simulink model "gtcs_math_v1"  (R2022b)
settings: Solver=VariableStepAuto  StartTime=0.0  StopTime=10  RelTol=1e-3
values from neighbouring files (symbols this model uses):
  B_load = 0.0047    [parameter_andar_servomotor.mat]
  B_motor = 0.00025    [parameter_andar_servomotor.mat]    (also in parameter_original_servomotor.mat)
  B_reducer = 0.001    [parameter_andar_servomotor.mat]
  GearRatio = 1    [parameter_andar_servomotor.mat]
  J_hysteresis_brake = 0.0016118    [parameter_andar_servomotor.mat]
  J_load = 0.0016118    [parameter_andar_servomotor.mat]
  J_motor = 0.0002548    [parameter_andar_servomotor.mat]    (also in parameter_original_servomotor.mat = 0.001)
  J_reducer = 1e-05    [parameter_andar_servomotor.mat]
  ke = 0.039313695    [parameter_andar_servomotor.mat]    (also in parameter_original_servomotor.mat = 0.04001501117)
  kt = 0.0378    [parameter_andar_servomotor.mat]    (also in parameter_original_servomotor.mat = 0.0375)
  L_motor = 6e-06    [parameter_andar_servomotor.mat]    (also in parameter_original_servomotor.mat = 3e-05)
  R_motor = 0.015    [parameter_andar_servomotor.mat]    (also in parameter_original_servomotor.mat = 0.075)
undefined symbols (not defined in the file or in its folder): sigbuilder_block
libraries: simulink x3, slpidlib x1
settings Model: DataDictionary=gtcs_math_v1.sldd  Creator=yusuf.ogut  LastModifiedBy=Yusuf
settings ModelReferenceCC: EnableRefExpFcnMdlSchedulingChecks=on

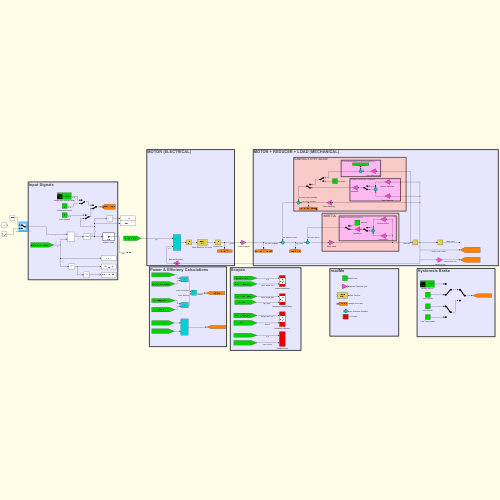
[thumbnail: Simulink's stored preview of the top-level diagram]
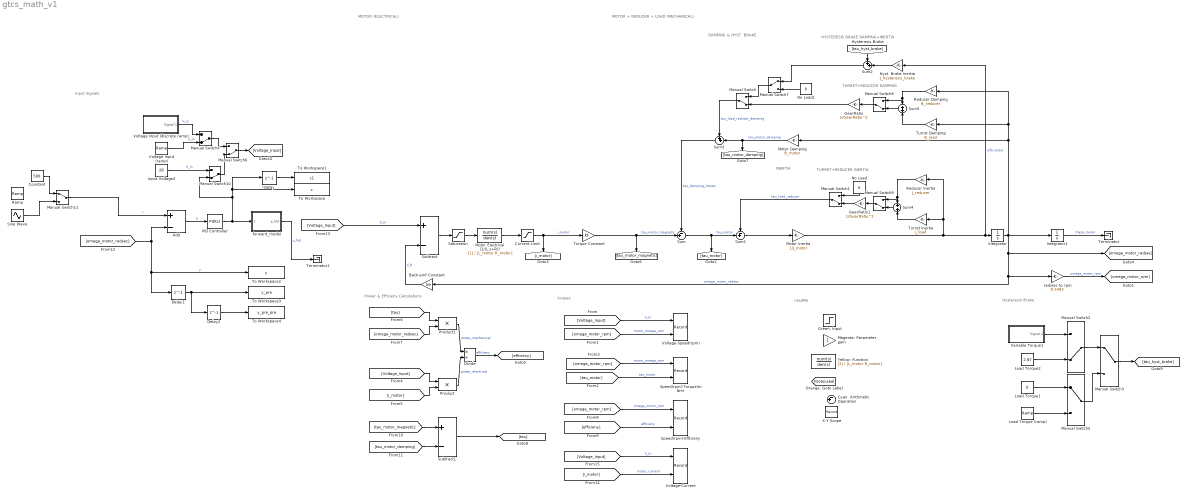
== system gtcs_math_v1 ==
  note: TURRET+REDUCER INERTIA
  note: TURRET+REDUCER DAMPING
  note: HYSTERESIS BRAKE DAMPING+INERTIA
  note: DAMPING & HYST. BRAKE
  note: INERTIA
  note: readMe
  note: MOTOR (ELECTRICAL)
  note: MOTOR + REDUCER + LOAD (MECHANICAL)
  note: Hysteresis Brake
  note: Input Signals
  note: Scopes
  note: Power & Efficieny Calculations
  Add : Sum  Inputs=+-
  Back-emf Constant : Gain  Gain=ke
  Constant : Constant  Value=500
  Current Limit : Saturate  UpperLimit=80  LowerLimit=-80
  Cyan: Arithmetic Operation : Sum  Inputs=-+|
  Delay : Delay  DelayLength=1  SampleTime=0.01
  Delay1 : Delay  DelayLength=1  SampleTime=0.01
  Delay2 : Delay  DelayLength=1  SampleTime=0.01
  Divide : Product  Inputs=*/
  GearRatio : Gain  Gain=1/GearRatio^2
  GearRatio1 : Gain  Gain=1/GearRatio^2
  Green: Input : Step  SampleTime=0
  Hyst. Brake Inertia : Gain  Gain=J_hysteresis_brake
  Input Voltage2 : Constant  Value=28
  Integrator : Integrator
  Integrator1 : Integrator
  Load Torque (ramp) : simulink/Sources/Ramp  slope=2.9/27  start=0  InitialOutput=1e-06
  Load Torque1 : Constant  Value=0
  Load Torque2 : Constant  Value=2.87
  "Magenta: Parameter, gain" : Gain
  Manual Switch{,1..2,4,6,8..10} (8 alike) : ManualSwitch  CurrentSetting=0
  Manual Switch{3,5,7,11} (4 alike) : ManualSwitch
  Motor Damping : Gain  Gain=B_motor
  Motor Electrical (1/(L.s+R)) : TransferFcn  Denominator=[L_motor R_motor]
  Motor Inertia : Gain  Gain=1/J_motor
  No Load : Constant  Value=0
  No Load1 : Constant  Value=0
  PID Controller : slpidlib/PID Controller  Controller=PID  Form=Parallel  TimeDomain=Continuous-time  UseExternalTs=off  SampleTime=-1  IntegratorMethod=Forward Euler  FilterMethod=Forward Euler  ControllerParametersSource=internal  P=1  I=1  UseKiTs=off  D=0  N=100  UseFilter=on  TunerSelectOption=Transfer Function Based (PID Tuner App)  InitialConditionSource=internal  InitialConditionForIntegrator=0  InitialConditionForFilter=0  DifferentiatorICPrevScaledInput=0  ExternalReset=none  TrackingMode=off  Kt=1  LimitOutput=off  SatLimitsSource=internal  UpperSaturationLimit=inf  LowerSaturationLimit=-inf  LinearizeAsGain=on  AntiWindupMode=none  Kb=1  LimitIntegrator=off  UpperIntegratorSaturationLimit=inf  LowerIntegratorSaturationLimit=-inf  POutMin=[]  POutMax=[]  IOutMin=[]  IOutMax=[]  DOutMin=[]  DOutMax=[]  NOutMin=[]  NOutMax=[]  SumOutMin=[]  SumOutMax=[]  SaturationOutMin=[]  SaturationOutMax=[]  PParamMin=[]  PParamMax=[]  IParamMin=[]  IParamMax=[]  DParamMin=[]  DParamMax=[]  NParamMin=[]  NParamMax=[]  KbParamMin=[]  KbParamMax=[]  KtParamMin=[]  KtParamMax=[]  KbOutMin=[]  KbOutMax=[]  KtOutMin=[]  KtOutMax=[]  IntegratorOutMin=[]  IntegratorOutMax=[]  FilterOutMin=[]  FilterOutMax=[]  SumI1OutMin=[]  SumI1OutMax=[]  SumI2OutMin=[]  SumI2OutMax=[]  SumI3OutMin=[]  SumI3OutMax=[]  SumI4OutMin=[]  SumI4OutMax=[]  SumDOutMin=[]  SumDOutMax=[]  DifferentiatorOutMin=[]  DifferentiatorOutMax=[]  FilterDiffOutCoefMin=[]  FilterDiffOutCoefMax=[]  ReciprocalOutMin=[]  ReciprocalOutMax=[]  SumDenOutMin=[]  SumDenOutMax=[]  SumNumOutMin=[]  SumNumOutMax=[]  DivideOutMin=[]  DivideOutMax=[]  UdiffTsProdOutMin=[]  UdiffTsProdOutMax=[]  NTsProdOutMin=[]  NTsProdOutMax=[]  UintegralTsProdOutMin=[]  UintegralTsProdOutMax=[]  UngainTsProdOutMin=[]  UngainTsProdOutMax=[]  ClampingZeroOutDataTypeStr=Inherit: Inherit via back propagation  ClampingZeroOutMin=[]  ClampingZeroOutMax=[]  FilterDenConstantOutDataTypeStr=Inherit: Inherit via back propagation  FilterDenConstantOutMin=[]  FilterDenConstantOutMax=[]  PCopyOutDataTypeStr=Inherit: Inherit via back propagation  PCopyOutMin=[]  PCopyOutMax=[]  NCopyOutDataTypeStr=Inherit: Inherit via back propagation  NCopyOutMin=[]  NCopyOutMax=[]  IntegratorContinuousStateAttributes=''  IntegratorStateMustResolveToSignalObject=off  IntegratorRTWStateStorageClass=Auto  FilterContinuousStateAttributes=''  FilterStateMustResolveToSignalObject=off  FilterRTWStateStorageClass=Auto  ParallelPVariant=InternalParameters  IdealPVariant=Disabled  IVariant=InternalParameters  DVariant=InternalParameters  IntegratorVariant=Continuous  SatVariant=Disabled  AWVariant=Passthrough  PCopyVariant=Disabled  TRVariant=Disabled  FdbkBlocksVariant=Forward  IdealPFdbkVariant=Disabled  SatFdbkVariant=Disabled  DerivativeFilterVariant=ContFilter  NVariant=InternalParameters  NCopyVariant=Disabled  FilterICVariant=InternalICsFilter  IntegratorICVariant=InternalICs  ExternalResetVariant=Disabled  TRSumVariant=Passthrough  SumFdbkVariant=Disabled  SumVariant=Sum_PID  TsampFilterVariant=InternalTs  TsampNgainVariant=Passthrough  TsampIntegralVariant=Passthrough  ExternalSaturationOutDataTypeStr=Inherit: Same as second input
  Product : Product
  Product1 : Product
  Ramp : simulink/Sources/Ramp  slope=25  start=0  InitialOutput=0
  Reducer Damping : Gain  Gain=B_reducer
  Reducer Inertia : Gain  Gain=J_reducer
  Saturation : Saturate  UpperLimit=28  LowerLimit=-28
  Sine Wave : Sin  Amplitude=400  SampleTime=0
  Speed(rpm)-Efficieny : Record  FileSettingsInternal="{\"entries\":[{\"content\":{\"excelSettings\":{\"content\":{},\"type\":\"Streamout.ExcelSettings\"}},\"type\":\"Streamout.FileSettingStorage\",\"uuid\":\"5ceb1766-4c77-4d68-bc5b-a68c05b999d6\"}],\"packageUris\":[\"http://schema.mathworks.com/mf0/streamout_blocks/R2020a\"],\"version\":\"1.0\"}"  Layout=[1 1]  SignalsInternal="{\"entries\":[{\"content\":{\"signals\":[{\"content\":{\"blockPath\":[\"gtcs_math_v1/Speed(rpm)-Efficieny\"],\"channel\":[],\"dimensions\":[1],\"domain\":\"gtcs_math_v1/Speed(rpm)-Efficieny\",\"lineColor\":\"#d95319\",\"plots\":[],\"port\":1,\"sid\":[],\"signalID\":761,\"signalName\":\"omega_motor_rpm\"},\"type\":\"RecordBlkView.Signal\",\"uuid\":\"6d182a02-5feb-48f3-9dd1-fc4c739d84c7\"},{\"content\":{\"blockPath\":[\"gtcs_math_v1/Speed(rpm)-Efficieny\"],\"channel\":[],\"dimensions\":[1],\"domain\":\"gtcs_math_v1/Speed(rpm)-Efficieny\",\"lineColor\":\"#edb120\",\"plots\":[],\"port\":2,\"sid\":[],\"signalID\":764,\"signalName\":\"efficieny\"},\"type\":\"RecordBlkView.Signal\",\"uuid\":\"5a7444f0-9e7b-4402-b735-20e3d0af58fb\"}]},\"type\":\"RecordBlkView.InputSignals\",\"uuid\":\"7a99b374-d198-444d-bc9b-5f1bb81e01e8\"}],\"packageUris\":[\"http://schema.mathworks.com/mf0/streamout_blocks/R2020a\"],\"version\":\"1.0\"}"  VisualizationBindings="{\"xyplotplugin\":{\"info\":[{\"series\":[],\"subplotID\":1}]}}"  CompatibilityTag=XY
  Speed(rpm)-Torque(mNm) : Record  FileSettingsInternal="{\"entries\":[{\"content\":{\"excelSettings\":{\"content\":{},\"type\":\"Streamout.ExcelSettings\"}},\"type\":\"Streamout.FileSettingStorage\",\"uuid\":\"fd18a3e1-7c27-470d-85cf-3c84a845ae30\"}],\"packageUris\":[\"http://schema.mathworks.com/mf0/streamout_blocks/R2020a\"],\"version\":\"1.0\"}"  Layout=[1 1]  SignalsInternal="{\"entries\":[{\"content\":{\"signals\":[{\"content\":{\"blockPath\":[\"gtcs_math_v1/Speed(rpm)-Torque(mNm)\"],\"channel\":[],\"dimensions\":[1],\"domain\":\"gtcs_math_v1/Speed(rpm)-Torque(mNm)\",\"lineColor\":\"#7e2f8e\",\"plots\":[],\"port\":1,\"sid\":[],\"signalID\":753,\"signalName\":\"motor_omega_rpm\"},\"type\":\"RecordBlkView.Signal\",\"uuid\":\"61d3b4c0-f085-4c37-bc40-0282be6f29b6\"},{\"content\":{\"blockPath\":[\"gtcs_math_v1/Speed(rpm)-Torque(mNm)\"],\"channel\":[],\"dimensions\":[1],\"domain\":\"gtcs_math_v1/Speed(rpm)-Torque(mNm)\",\"lineColor\":\"#77ac30\",\"plots\":[],\"port\":2,\"sid\":[],\"signalID\":756,\"signalName\":\"tau_motor\"},\"type\":\"RecordBlkView.Signal\",\"uuid\":\"cfa706d7-1d71-4160-89ad-7ed0bbc03a52\"}]},\"type\":\"RecordBlkView.InputSignals\",\"uuid\":\"81d05471-cab0-4422-b169-8359f553d494\"}],\"packageUris\":[\"http://schema.mathworks.com/mf0/streamout_blocks/R2020a\"],\"version\":\"1.0\"}"  VisualizationBindings="{\"xyplotplugin\":{\"info\":[{\"series\":[],\"subplotID\":1}]}}"  CompatibilityTag=XY
  Subtract : Sum  Inputs=+-
  Subtract1 : Sum  Inputs=+-
  Sum : Sum  Inputs=-+|
  Sum1 : Sum  Inputs=-+|
  Sum2 : Sum  Inputs=++|
  Sum3 : Sum  Inputs=++|
  Sum4 : Sum
  Sum5 : Sum
  Terminator : Terminator
  Terminator1 : Terminator
  To Workspace : ToWorkspace  VariableName=c  SampleTime=0.01
  To Workspace1 : ToWorkspace  VariableName=c1  SampleTime=0.01
  To Workspace2 : ToWorkspace  VariableName=y  SampleTime=0.01
  To Workspace3 : ToWorkspace  VariableName=y_pre  SampleTime=0.01
  To Workspace4 : ToWorkspace  VariableName=y_pre_pre  SampleTime=0.01
  Torque Constant : Gain  Gain=kt
  Turret Damping : Gain  Gain=B_load
  Turret Inertia : Gain  Gain=J_load
  Variable Torque1 : Subsystem  Tag=STV Subsys  LoadFcn=sigbuilder_block('load');  StartFcn=sigbuilder_block('start');  StopFcn=sigbuilder_block('stop');  ClipboardFcn=sigbuilder_block('clipboard');  mask(Sigbuilder block){tuvar=[0:10]}
      mask help: Simulink:masks:SigbuilderBlock_MD
      mask init:
      | if ~strcmp(get_param(bdroot(gcbh),'SimulationStatus'),'stopped') tuvar = sigbuilder_block('maskInit'); end
      settings: CopyFcn=sigbuilder_block('copy');  DeleteFcn=sigbuilder_block('delete');  ModelCloseFcn=sigbuilder_block('modelClose');  PreSaveFcn=sigbuilder_block('preSave');  PauseFcn=sigbuilder_block('pause');  ContinueFcn=sigbuilder_block('continue');  NameChangeFcn=sigbuilder_block('namechange');  OpenFcn=sigbuilder_block('open',[0 36 1440 716.25 ]);  CloseFcn=sigbuilder_block('close');
      mask Display: plot(0, 0, 100, 100,[2, 2, 32, 32, 2], [68, 8, 8, 68, 68],[32, 2], [38, 38], [32, 19, 2],[53, 60, 44], [32, 17, 17, 2],[16, 16, 31, 31]);txt = getActiveGroup(gcbh);text(2, 100, txt,'verticalAlignment', 'top');
  Voltage Input (discrete ramp) : Subsystem  Tag=STV Subsys  LoadFcn=sigbuilder_block('load');  StartFcn=sigbuilder_block('start');  StopFcn=sigbuilder_block('stop');  ClipboardFcn=sigbuilder_block('clipboard');  mask(Sigbuilder block){tuvar=[0:10]}
      mask help: Simulink:masks:SigbuilderBlock_MD
      mask init:
      | if ~strcmp(get_param(bdroot(gcbh),'SimulationStatus'),'stopped') tuvar = sigbuilder_block('maskInit'); end
      settings: CopyFcn=sigbuilder_block('copy');  DeleteFcn=sigbuilder_block('delete');  ModelCloseFcn=sigbuilder_block('modelClose');  PreSaveFcn=sigbuilder_block('preSave');  PauseFcn=sigbuilder_block('pause');  ContinueFcn=sigbuilder_block('continue');  NameChangeFcn=sigbuilder_block('namechange');  OpenFcn=sigbuilder_block('open',[0.75 36.75 718.5 709.5 ]);  CloseFcn=sigbuilder_block('close');
      mask Display: plot(0, 0, 100, 100,[2, 2, 32, 32, 2], [68, 8, 8, 68, 68],[32, 2], [38, 38], [32, 19, 2],[53, 60, 44], [32, 17, 17, 2],[16, 16, 31, 31]);txt = getActiveGroup(gcbh);text(2, 100, txt,'verticalAlignment', 'top');
  Voltage Input (ramp) : simulink/Sources/Ramp  slope=0.5  start=50  InitialOutput=5
  Voltage-Current : Record  FileSettingsInternal="{\"entries\":[{\"content\":{\"excelSettings\":{\"content\":{},\"type\":\"Streamout.ExcelSettings\"}},\"type\":\"Streamout.FileSettingStorage\",\"uuid\":\"c1f11984-e9ff-41c6-9b03-641b67f8d55f\"}],\"packageUris\":[\"http://schema.mathworks.com/mf0/streamout_blocks/R2020a\"],\"version\":\"1.0\"}"  Layout=[1 1]  SignalsInternal="{\"entries\":[{\"content\":{\"signals\":[{\"content\":{\"blockPath\":[\"gtcs_math_v1/Voltage-Current\"],\"channel\":[],\"dimensions\":[1],\"domain\":\"gtcs_math_v1/Voltage-Current\",\"lineColor\":\"#64d413\",\"plots\":[],\"port\":1,\"sid\":[],\"signalID\":737,\"signalName\":\"V_in\"},\"type\":\"RecordBlkView.Signal\",\"uuid\":\"6bf1e316-3e80-4ccb-9077-63da5d7ffe28\"},{\"content\":{\"blockPath\":[\"gtcs_math_v1/Voltage-Current\"],\"channel\":[],\"dimensions\":[1],\"domain\":\"gtcs_math_v1/Voltage-Current\",\"lineColor\":\"#ff13a6\",\"plots\":[],\"port\":2,\"sid\":[],\"signalID\":740,\"signalName\":\"motor_current\"},\"type\":\"RecordBlkView.Signal\",\"uuid\":\"9848fcd3-6a94-4634-a870-fd3925440432\"}]},\"type\":\"RecordBlkView.InputSignals\",\"uuid\":\"0598c337-9d6d-44b8-8272-d3ed3f6b23dd\"}],\"packageUris\":[\"http://schema.mathworks.com/mf0/streamout_blocks/R2020a\"],\"version\":\"1.0\"}"  VisualizationBindings="{\"xyplotplugin\":{\"info\":[{\"series\":[],\"subplotID\":1}]}}"  CompatibilityTag=XY
  Voltage-Speed(rpm) : Record  FileSettingsInternal="{\"entries\":[{\"content\":{\"excelSettings\":{\"content\":{},\"type\":\"Streamout.ExcelSettings\"}},\"type\":\"Streamout.FileSettingStorage\",\"uuid\":\"59ffcc84-2ca6-4e0b-9cea-5daa768fe9a7\"}],\"packageUris\":[\"http://schema.mathworks.com/mf0/streamout_blocks/R2020a\"],\"version\":\"1.0\"}"  Layout=[1 1]  SignalsInternal="{\"entries\":[{\"content\":{\"signals\":[{\"content\":{\"blockPath\":[\"gtcs_math_v1/Voltage-Speed(rpm)\"],\"channel\":[],\"dimensions\":[1],\"domain\":\"gtcs_math_v1/Voltage-Speed(rpm)\",\"lineColor\":\"#fe330a\",\"plots\":[],\"port\":1,\"sid\":[],\"signalID\":729,\"signalName\":\"V_in\"},\"type\":\"RecordBlkView.Signal\",\"uuid\":\"0be176e8-9078-4797-8299-9f8d682af79f\"},{\"content\":{\"blockPath\":[\"gtcs_math_v1/Voltage-Speed(rpm)\"],\"channel\":[],\"dimensions\":[1],\"domain\":\"gtcs_math_v1/Voltage-Speed(rpm)\",\"lineColor\":\"#22b573\",\"plots\":[],\"port\":2,\"sid\":[],\"signalID\":732,\"signalName\":\"motor_omega_rpm\"},\"type\":\"RecordBlkView.Signal\",\"uuid\":\"08d827e7-7879-480f-bd38-e635a1023ee3\"}]},\"type\":\"RecordBlkView.InputSignals\",\"uuid\":\"bea77a8c-dea2-49d2-ad1a-3d36c4badb96\"}],\"packageUris\":[\"http://schema.mathworks.com/mf0/streamout_blocks/R2020a\"],\"version\":\"1.0\"}"  VisualizationBindings="{\"xyplotplugin\":{\"info\":[{\"series\":[],\"subplotID\":1}]}}"  CompatibilityTag=XY
  X-Y Scope : Record  FileSettingsInternal="{\"entries\":[{\"content\":{\"excelSettings\":{\"content\":{},\"type\":\"Streamout.ExcelSettings\"}},\"type\":\"Streamout.FileSettingStorage\",\"uuid\":\"943fa2fc-e112-4a03-8195-d1d29e8222db\"}],\"packageUris\":[\"http://schema.mathworks.com/mf0/streamout_blocks/R2020a\"],\"version\":\"1.0\"}"  Layout=[1 1]  SignalsInternal="{\"entries\":[{\"content\":{\"signals\":[{\"content\":{\"blockPath\":[\"gtcs_math_v1/X-Y Scope\"],\"channel\":[],\"dimensions\":[1],\"domain\":\"gtcs_math_v1/X-Y Scope\",\"lineColor\":\"#7e2f8e\",\"plots\":[],\"port\":1,\"sid\":[],\"signalID\":745},\"type\":\"RecordBlkView.Signal\",\"uuid\":\"e93512a9-84e9-4859-a5ce-8b5415996e34\"},{\"content\":{\"blockPath\":[\"gtcs_math_v1/X-Y Scope\"],\"channel\":[],\"dimensions\":[1],\"domain\":\"gtcs_math_v1/X-Y Scope\",\"lineColor\":\"#77ac30\",\"plots\":[],\"port\":2,\"sid\":[],\"signalID\":748},\"type\":\"RecordBlkView.Signal\",\"uuid\":\"f7652492-03bf-4964-8f75-b0621181aa5a\"}]},\"type\":\"RecordBlkView.InputSignals\",\"uuid\":\"007b276a-6083-418b-9662-27ae14b522bb\"}],\"packageUris\":[\"http://schema.mathworks.com/mf0/streamout_blocks/R2020a\"],\"version\":\"1.0\"}"  VisualizationBindings="{\"xyplotplugin\":{\"info\":[{\"series\":[],\"subplotID\":1}]}}"  CompatibilityTag=XY
  Yellow: Function : TransferFcn  Denominator=[L_motor R_motor]
  forward_model : MATLAB Function  TreatAsAtomicUnit=on
  rad/sec to rpm : Gain  Gain=9.5493
  wires:
  Subtract/1 -> Saturation/1
  Torque Constant/1 -> Sum/2, [tau_motor_magnetic]  "tau_motor_magnetic"
  Motor Inertia/1 -> Hyst. Brake Inertia/1, Integrator/1, Turret Inertia/1, Reducer Inertia/1  "alfa motor"
  Integrator/1 -> Integrator1/1, [omega_motor_radsec], rad/sec to rpm/1, Back-emf Constant/1, Turret Damping/1, Reducer Damping/1, Motor Damping/1  "omega_motor_radsec"
  Integrator1/1 -> Terminator/1  "theta_motor"
  rad/sec to rpm/1 -> [omega_motor_rpm]  "omega_motor_rpm"
  Motor Electrical (1/(L.s+R))/1 -> Current Limit/1
  [Voltage_Input] -> Subtract/1  "V_in"
  [Voltage_Input] -> Voltage-Speed(rpm)/1  "V_in"
  [omega_motor_rpm] -> Voltage-Speed(rpm)/2  "motor_omega_rpm"
  [omega_motor_rpm] -> Speed(rpm)-Torque(mNm)/1  "motor_omega_rpm"
  [tau_motor] -> Speed(rpm)-Torque(mNm)/2  "tau_motor"
  [omega_motor_rpm] -> Speed(rpm)-Efficieny/1  "omega_motor_rpm"
  [efficieny] -> Speed(rpm)-Efficieny/2  "efficieny"
  Product1/1 -> Divide/1  "power_mechanical"
  Product/1 -> Divide/2  "power_electrical"
  [i_motor] -> Product/2
  [omega_motor_radsec] -> Product1/2
  [tau] -> Product1/1
  Divide/1 -> [efficieny]  "efficieny"
  [Voltage_Input] -> Product/1
  Current Limit/1 -> Torque Constant/1, [i_motor]  "i_motor"
  Saturation/1 -> Motor Electrical (1/(L.s+R))/1
  Motor Damping/1 -> [tau_motor_damping], Sum3/2  "tau_motor_damping"
  Sum1/1 -> Motor Inertia/1
  Sum/1 -> Sum1/2, [tau_motor]  "tau_motor"
  [tau_motor_magnetic] -> Subtract1/1
  [tau_motor_damping] -> Subtract1/2
  Subtract1/1 -> [tau]
  Turret Inertia/1 -> Sum4/2
  Manual Switch1/1 -> Sum1/1  "tau_load_reducer"
  Variable Torque1/1(Signal 1) -> Manual Switch2/1
  Load Torque2/1 -> Manual Switch2/2
  Manual Switch2/1 -> Manual Switch3/1
  Manual Switch3/1 -> [tau_hyst_brake]
  Voltage Input (discrete ramp)/1(Signal 1) -> Manual Switch4/1  "V_in"
  Voltage Input (ramp)/1 -> Manual Switch4/2  "V_in"
  Input Voltage2/1 -> Manual Switch10/1  "V_in"
  Manual Switch4/1 -> Manual Switch6/1
  Manual Switch6/1 -> [Voltage_Input]
  Manual Switch/1 -> Sum3/1  "tau_load_reducer_damping"
  Sum3/1 -> Sum/1  "tau_damping_losses"
  Load Torque (ramp)/1 -> Manual Switch5/2
  Load Torque1/1 -> Manual Switch5/1
  Manual Switch5/1 -> Manual Switch3/2
  [Voltage_Input] -> Voltage-Current/1  "V_in"
  [i_motor] -> Voltage-Current/2  "motor_current"
  Reducer Inertia/1 -> Manual Switch9/1, Sum4/1
  GearRatio1/1 -> Manual Switch1/2
  No Load/1 -> Manual Switch1/1
  Reducer Damping/1 -> Manual Switch8/1, Sum5/1
  Turret Damping/1 -> Sum5/2
  GearRatio/1 -> Manual Switch/2
  No Load1/1 -> Manual Switch7/2
  Manual Switch7/1 -> Manual Switch/1
  Sum5/1 -> Manual Switch8/2
  Manual Switch8/1 -> GearRatio/1
  Sum4/1 -> Manual Switch9/2
  Manual Switch9/1 -> GearRatio1/1
  [tau_hyst_brake] -> Sum2/1
  Hyst. Brake Inertia/1 -> Sum2/2
  Sum2/1 -> Manual Switch7/1
  [omega_motor_radsec] -> To Workspace2/1, Delay1/1, Add/2  "y"
  Add/1 -> PID Controller/1  "e"
  PID Controller/1 -> forward_model/1(c), Delay/1, To Workspace/1, Manual Switch10/2  "c"
  Manual Switch10/1 -> Manual Switch6/2
  Sine Wave/1 -> Manual Switch11/2
  Manual Switch11/1 -> Add/1  "r"
  Back-emf Constant/1 -> Subtract/2  "V_b"
  forward_model/1(y_hat) -> Terminator1/1  "y_hat"
  Delay/1 -> To Workspace1/1
  Delay1/1 -> Delay2/1, To Workspace3/1
  Delay2/1 -> To Workspace4/1
  Constant/1 -> Manual Switch11/1

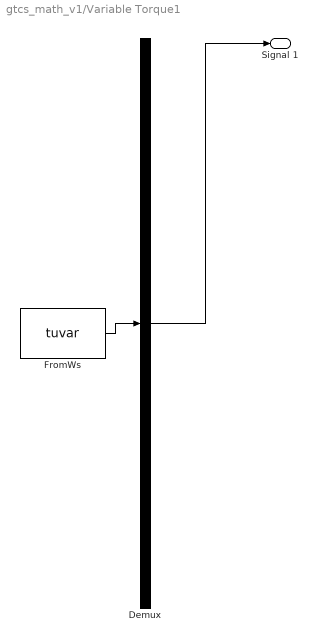
== system gtcs_math_v1/Variable Torque1 ==
  Demux : Demux  Tag=STV Demux  Outputs=1
      settings: DisplayOption=none
  FromWs : FromWorkspace  Tag=STV FromWs  VariableName=tuvar
      SigBuilderData=|
      | common.afterFinalStr = 'Extrapolate'
      | common.sampleTime = 0
      | dataSet.timeRange = [0 30]
      | dataSet.name = 'Group 1'
      | sbobj.Groups.Name = 'Group 1'
      | sbobj.Groups.Signals.Name = 'Signal 1'
      | sbobj.Groups.Signals.XData = [0 2 2 6 6 10 10 15 15 30]
      | sbobj.Groups.Signals.YData = [0 0 1 1 2 2 2.5 2.5 3 3]
      | sbobj.Groups.TimeRange = [0 30]
  Signal 1 : Outport  Tag=STV Outport
  wires:
  Demux/1 -> Signal 1/1
  FromWs/1 -> Demux/1

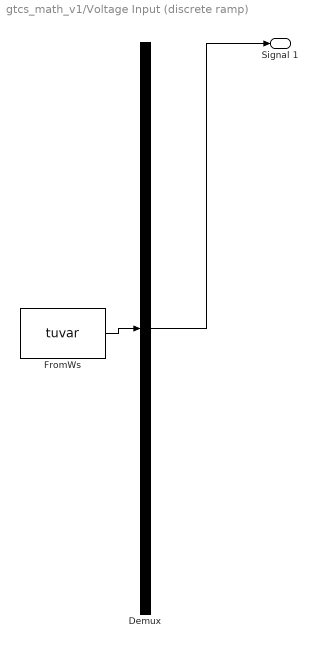
== system gtcs_math_v1/Voltage Input (discrete ramp) ==
  Demux : Demux  Tag=STV Demux  Outputs=1
      settings: DisplayOption=none
  FromWs : FromWorkspace  Tag=STV FromWs  VariableName=tuvar
      SigBuilderData=|
      | common.afterFinalStr = 'Extrapolate'
      | common.sampleTime = 0
      | dataSet.timeRange = [0 34]
      | dataSet.name = 'Group 1'
      | sbobj.Groups.Name = 'Group 1'
      | sbobj.Groups.Signals.Name = 'Signal 1'
      | sbobj.Groups.Signals.XData = [0 8 10 12 14 16 18 20 22 24 26 28 30 32 34]
      | sbobj.Groups.Signals.YData = [0 3.27 3.27 7.28 7.28 11.23 11.23 15.19 15.19 19.17 19.17 23.18 23.18 32 32]
      | sbobj.Groups.TimeRange = [0 34]
  Signal 1 : Outport  Tag=STV Outport
  wires:
  FromWs/1 -> Demux/1
  Demux/1 -> Signal 1/1

== matlab function gtcs_math_v1/forward_model ==
  data: c input; y_hat output
function y_hat = fcn(c)
    Phi = [0.3935   21.8693    0.4187   -0.7620    0.5025    0.0944;
          -0.3620   21.9286    0.5094   -0.0033   -0.4898   -0.7228;
           0.9043   20.7120   -0.4479    0.9195    0.0119   -0.7014;
          -0.9273   21.3178    0.3594   -0.3192    0.3982   -0.4850;
          -0.1187   21.2294    0.3102    0.1705    0.7818    0.6814;
          10.0202    8.5052   14.6225    7.6127   12.1964    6.3142];
    BIAS = -1;
    % FORWARD PASS:
    NUM_INP = 1; NUM_HID = 5;
    input_vector = [c;BIAS];
    S1 = Phi(1:NUM_HID,1:NUM_INP+1)*input_vector;
    O1 = tanh(S1);
    S2 = Phi(NUM_HID+1:end,1:NUM_HID+1)*[O1;BIAS];
    y_hat =S2;
end
